simulink model "Initial_Pose"  (R2022b)
settings: Solver=FixedStepDiscrete  StartTime=0.0  StopTime=inf  FixedStep=0.001  RelTol=1e-3  EnableMultiTasking=on
PreLoadFcn:
  | set_param(gcs, 'RTWSystemTargetFile', 'franka_emika_panda.tlc');
  | init_Initial_Pose();
libraries: franka_simulink_library x5, simulink x1
settings Model: SimulationMode=external  ExtModeTrigDuration=10000  Creator=vasi_ko  LastModifiedBy=host
settings SolverCC: AlgebraicLoopSolver=TrustRegion
settings DataIOCC: LimitDataPoints=on  SaveFormat=Array  ReturnWorkspaceOutputs=off
settings OptimizationCC: DefaultParameterBehavior=Inlined  EnhancedBackFolding=on  PassReuseOutputArgsThreshold=0  OptimizeBlockOrder=speed  DifferentSizesBufferReuse=on  OptimizationCustomize=off
settings DebuggingCC: SolverPrmCheckMsg=warning  ParameterTunabilityLossMsg=error  UnconnectedInputMsg=warning  UnconnectedOutputMsg=warning  UnconnectedLineMsg=warning  SFUnexpectedBacktrackingDiag=warning  SFNoUnconditionalDefaultTransitionDiag=warning  SFExecutionAtInitializationDiag=none  SFMachineParentedDataDiag=warning  ArithmeticOperatorsInVariantConditions=warning
settings HardwareCC: ProdBitPerLong=64  ProdHWDeviceType=Intel->x86-64 (Linux 64)
settings ModelReferenceCC: EnableRefExpFcnMdlSchedulingChecks=on  PropagateSignalLabelsOutOfModel=off
settings SFSimCC: SimUseLocalCustomCode=off  MATLABDynamicMemAlloc=off  CustomCodeUndefinedFunction=UseInterfaceOnly  SimTargetLang=C++
settings RTWCC: SystemTargetFile=franka_emika_panda.tlc  RTWVerbose=off  RTWUseLocalCustomCode=off  Toolchain=Franka Simulink | gmake (64-bit linux)  BuildConfiguration=Faster Runs  TargetLang=C++  DLArmComputeVersion=19.05
settings CodeAppCC: ForceParamTrailComments=on  OperatorAnnotations=on
settings STFCustomTargetCC: TargetLangStandard=C99 (ISO)  ModelReferenceCompliant=off  MatFileLogging=on  GRTInterface=on  UseToolchainInfoCompliant=on  SystemTargetFile=franka_emika_panda.tlc
settings GRTTargetCC: ModelReferenceCompliant=off  ParMdlRefBuildCompliant=off  CompOptLevelCompliant=off  ConcurrentExecutionCompliant=off  CombineOutputUpdateFcns=off  CPPClassGenCompliant=off  GRTInterface=on  ExtModeStaticAlloc=on  ExtModeTransport=1  ExtModeMexFile=ext_xcp  ExtModeIntrfLevel=Level2 - Open
settings ConfigComp: CovMetricSettings=dw  CovSaveCumulativeToWorkspaceVar=on  CovSaveSingleToWorkspaceVar=on  CovExternalEMLEnable=off  CovSFcnEnable=off

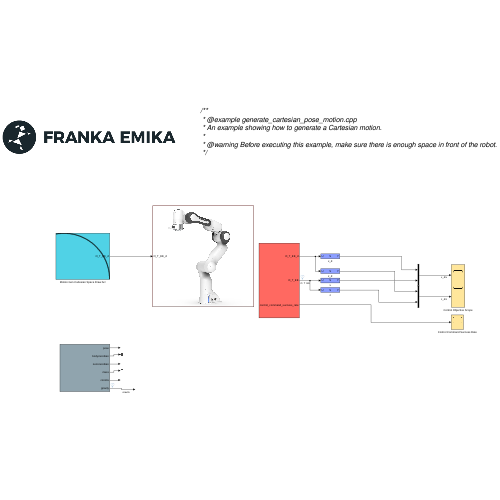
[thumbnail: Simulink's stored preview of the top-level diagram]
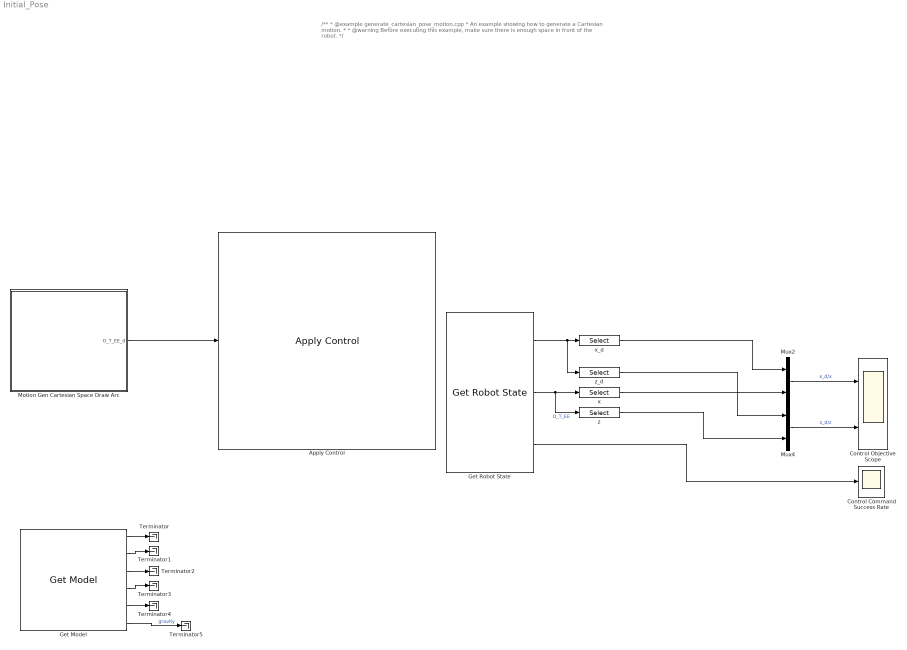
== system Initial_Pose ==
  note: /**
      |  * @example generate_cartesian_pose_motion.cpp
      |  * An example showing how to generate a Cartesian motion.
      |  *
      |  * @warning Before executing this example, make sure there is enough space in front of the robot.
      |  */
  Apply Control : franka_simulink_library/Apply Control  robot_ip=robot_ip  gripper_attached=off  control_mode=Cartesian Pose - Internal Controller Mode  controller_choice=Joint Impedance Controller  elbow_control=off  collision_thresholds=100*ones(1,52)  joint_impedance=[3000, 3000, 3000, 2500, 2500, 2000, 2000]  cartesian_impedance=cartesian_impedance  load_inertia=load_inertia  EE_T_K=EE_T_K  init_joint_configuration_req=on  init_joint_configuration=q_init
      settings: SourceProductName=Franka Emika Simulink Support Package
  Control Command Success Rate : Scope
  Control Objective Scope : Scope  NumInputPorts=2
  Get Model : franka_simulink_library/Get Model  robot_ip=robot_ip
      settings: SourceProductName=Franka Emika Simulink Support Package
  Get Robot State : franka_simulink_library/Get Robot State  robot_ip=robot_ip  signals_requested='O_T_EE_d O_T_EE control_command_success_rate'
      settings: SourceProductName=Franka Emika Simulink Support Package
  Motion Gen Cartesian Space Draw Arc : Subsystem
      mask Display:
      | pos = get_param(gcb, 'Position');
      | width = pos(3) - pos(1);
      | x = [0:width];
      | y = sin(x/180*pi);
      | % Parameters 'm' and 'b' must be defined in 'Parameters & Dialog' pane.
      | plot(cos(x/180*pi*0.5), sin(x/180*pi*0.5));
      | 
      | port_label('output',1,'O_T_EE_d');
  Mux2 : Mux  Inputs=2
  Mux4 : Mux  Inputs=2
  Terminator{,1..5} (6 alike) : Terminator
  x : Selector  InputPortWidth=16  IndexOptions=Index vector (dialog)  Indices=13  OutputSizes=1
  x_d : Selector  InputPortWidth=16  IndexOptions=Index vector (dialog)  Indices=13  OutputSizes=1
  z : Selector  InputPortWidth=16  IndexOptions=Index vector (dialog)  Indices=15  OutputSizes=1
  z_d : Selector  InputPortWidth=16  IndexOptions=Index vector (dialog)  Indices=15  OutputSizes=1
  wires:
  x/1 -> Mux2/2
  z/1 -> Mux4/2
  Mux2/1 -> Control Objective Scope/1  "x_d/x"
  Mux4/1 -> Control Objective Scope/2  "z_d/z"
  Get Robot State/1 -> z_d/1, x_d/1
  x_d/1 -> Mux2/1
  Motion Gen Cartesian Space Draw Arc/1(O_T_EE_d) -> Apply Control/1
  z_d/1 -> Mux4/1
  Get Robot State/2 -> z/1, x/1  "O_T_EE"
  Get Robot State/3 -> Control Command Success Rate/1
  Get Model/1 -> Terminator/1
  Get Model/2 -> Terminator1/1
  Get Model/3 -> Terminator2/1
  Get Model/4 -> Terminator3/1
  Get Model/5 -> Terminator4/1
  Get Model/6 -> Terminator5/1  "gravity"

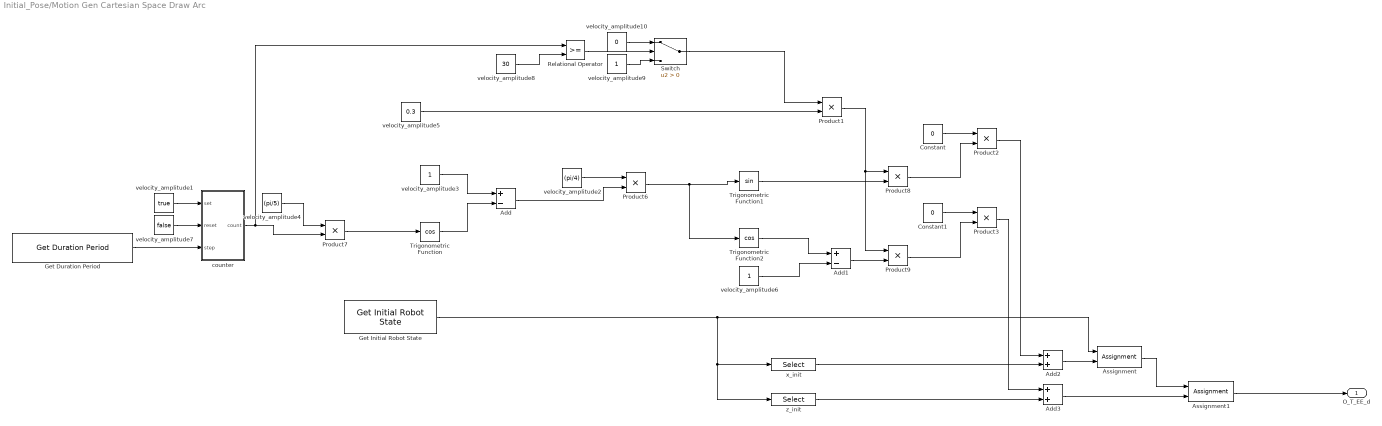
== system Initial_Pose/Motion Gen Cartesian Space Draw Arc ==
  Add : Sum  Inputs=+-
  Add1 : Sum  Inputs=+-
  Add2 : Sum
  Add3 : Sum
  Assignment : Assignment  DiagnosticForDimensions=Warning  IndexOptions=Index vector (dialog)  Indices=13  OutputSizes=1
  Assignment1 : Assignment  DiagnosticForDimensions=Warning  IndexOptions=Index vector (dialog)  Indices=15  OutputSizes=1
  Constant : Constant  Value=0
  Constant1 : Constant  Value=0
  Get Duration Period : franka_simulink_library/Get Duration Period  robot_ip=robot_ip
      settings: SourceProductName=Franka Emika Simulink Support Package
  Get Initial Robot State : franka_simulink_library/Get Initial Robot State  robot_ip=robot_ip  signals_requested='O_T_EE_c'
      settings: SourceProductName=Franka Emika Simulink Support Package
  Product{1..3,6..9} (7 alike) : Product
  Relational Operator : RelationalOperator  OutDataTypeStr=boolean  InputSameDT=off
  Switch : Switch  Criteria=u2 > Threshold  SaturateOnIntegerOverflow=off  InputSameDT=off
  Trigonometric Function : Trigonometry  Operator=cos  NumberOfIterations=50
  Trigonometric Function1 : Trigonometry  NumberOfIterations=50
  Trigonometric Function2 : Trigonometry  Operator=cos
  counter : Subsystem
  velocity_amplitude1 : Constant  Value=true  VectorParams1D=off
  velocity_amplitude10 : Constant  Value=0  VectorParams1D=off
  velocity_amplitude2 : Constant  Value=(pi/4)  VectorParams1D=off
  velocity_amplitude3 : Constant  VectorParams1D=off
  velocity_amplitude4 : Constant  Value=(pi/5)  VectorParams1D=off
  velocity_amplitude5 : Constant  Value=0.3  VectorParams1D=off
  velocity_amplitude6 : Constant  VectorParams1D=off
  velocity_amplitude7 : Constant  Value=false  VectorParams1D=off
  velocity_amplitude8 : Constant  Value=30  VectorParams1D=off
  velocity_amplitude9 : Constant  VectorParams1D=off
  x_init : Selector  InputPortWidth=16  IndexOptions=Index vector (dialog)  Indices=13  OutputSizes=1
  z_init : Selector  InputPortWidth=16  IndexOptions=Index vector (dialog)  Indices=15  OutputSizes=1
  O_T_EE_d : Outport  VectorParamsAs1DForOutWhenUnconnected=off
  wires:
  Product8/1 -> Product2/2
  x_init/1 -> Add2/2
  Assignment/1 -> Assignment1/1
  Add2/1 -> Assignment/2
  Get Initial Robot State/1 -> z_init/1, x_init/1, Assignment/1
  velocity_amplitude2/1 -> Product6/1
  velocity_amplitude3/1 -> Add/1
  velocity_amplitude4/1 -> Product7/1
  Trigonometric Function/1 -> Add/2
  Product7/1 -> Trigonometric Function/1
  Add/1 -> Product6/2
  Product6/1 -> Trigonometric Function1/1, Trigonometric Function2/1
  Trigonometric Function1/1 -> Product8/2
  Trigonometric Function2/1 -> Add1/1
  velocity_amplitude6/1 -> Add1/2
  Add1/1 -> Product9/2
  velocity_amplitude5/1 -> Product1/2
  Switch/1 -> Product1/1
  Product1/1 -> Product9/1, Product8/1
  Add3/1 -> Assignment1/2
  Get Duration Period/1 -> counter/3(step)
  velocity_amplitude1/1 -> counter/1(set)
  velocity_amplitude7/1 -> counter/2(reset)
  counter/1(count) -> Relational Operator/1, Product7/2
  Assignment1/1 -> O_T_EE_d/1
  z_init/1 -> Add3/2
  velocity_amplitude8/1 -> Relational Operator/2
  Relational Operator/1 -> Switch/2
  velocity_amplitude9/1 -> Switch/3
  velocity_amplitude10/1 -> Switch/1
  Constant/1 -> Product2/1
  Product2/1 -> Add2/1
  Constant1/1 -> Product3/1
  Product9/1 -> Product3/2
  Product3/1 -> Add3/1

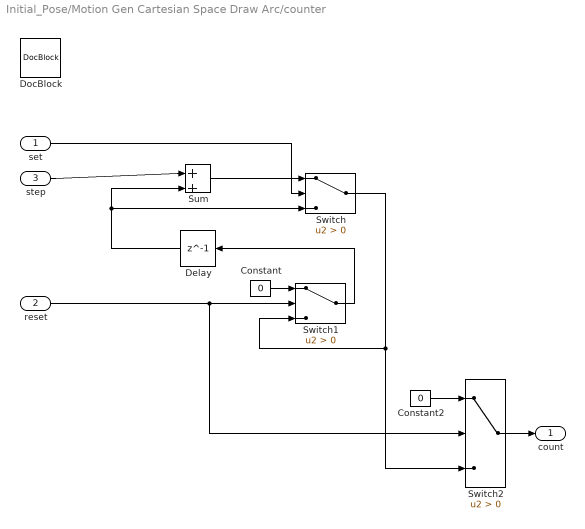
== system Initial_Pose/Motion Gen Cartesian Space Draw Arc/counter ==
  set : Inport  OutDataTypeStr=boolean
  reset : Inport  Port=2  OutDataTypeStr=boolean
  step : Inport  Port=3  OutDataTypeStr=double
  Constant : Constant  Value=0  OutDataTypeStr=double
  Constant2 : Constant  Value=0  OutDataTypeStr=double
  Delay : Delay  DelayLength=1  InitialCondition=0
  DocBlock : simulink/Model-Wide Utilities/DocBlock  DocumentType=Text
      content=|
      | %% counter
      | %
      | % This library includes the counter functionality that increases
      | % it's output by an input step factor for each computational step. The counter
      | % can also be externaly reset.
      | % -----------------------------------------------------------------------
      | % Author    : Konstantinos Vasios
      | % Date      : 01.09.2017
      | % Copyright : Franka Emika GmbH
      | % -----------------------------------------------------------------------
      | %
      | % Inputs:
      | % @param set : activates the counter. (data type: boolean, dimension: 1)
      | % @param reset: it resets the counter. Count starts from 0. (data type: boolean, dimension: 1)
      | % @param step: increment factor. (data type: real, dimension: 1)
      | %
      | % Outputs:
      | % @return count: current counter value. (data type: real, dimension: 1)
      | %% -----------------------------------------------------------------------
  Sum : Sum  Inputs=|++
  Switch : Switch  Criteria=u2 > Threshold  SaturateOnIntegerOverflow=off  InputSameDT=off
  Switch1 : Switch  Criteria=u2 > Threshold  OutDataTypeStr=double  SaturateOnIntegerOverflow=off  InputSameDT=off
  Switch2 : Switch  Criteria=u2 > Threshold  OutDataTypeStr=double  SaturateOnIntegerOverflow=off  InputSameDT=off
  count : Outport  OutDataTypeStr=double  VectorParamsAs1DForOutWhenUnconnected=off
  wires:
  Switch1/1 -> Delay/1
  Constant/1 -> Switch1/1
  reset/1 -> Switch2/2, Switch1/2
  Delay/1 -> Switch/3, Sum/2
  step/1 -> Sum/1
  Switch/1 -> Switch2/3, Switch1/3
  set/1 -> Switch/2
  Sum/1 -> Switch/1
  Constant2/1 -> Switch2/1
  Switch2/1 -> count/1
